simulink subsystem "AeroPropRef"  (R2024a)
settings: Solver=VariableStepAuto  StartTime=0.0  StopTime=10.0  RelTol=1e-3
undefined symbols (not defined in the file): Force_b, Fprop_r, H_b, Hdot_b, Moment_b, Mprop_r, SimIn, SimPar
libraries: starslibAxisTransformations x2, libAxisTransformations x2
settings Model: Creator=drhill  LastModifiedBy=azmol
settings SolverCC: AlgebraicLoopSolver=TrustRegion
settings OptimizationCC: ReuseModelBlockBuffer=off
settings DebuggingCC: UnconnectedInputMsg=warning  UnconnectedOutputMsg=warning  UnconnectedLineMsg=warning
settings ModelReferenceCC: EnableRefExpFcnMdlSchedulingChecks=on
settings RTWCC: GPUComputeCapability=3.5  DLArmComputeVersion=19.05

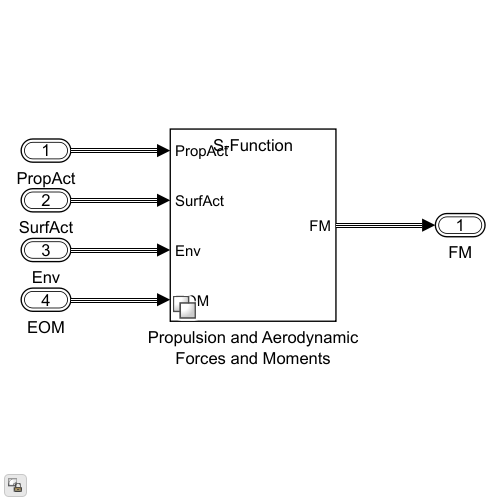
[thumbnail: Simulink's stored preview of the top-level diagram]
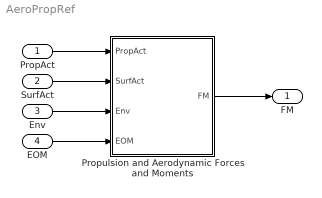
== system AeroPropRef ==
  PropAct : Inport  OutDataTypeStr=Bus: BUS_PROP_ACTUATOR
  SurfAct : Inport  Port=2  OutDataTypeStr=Bus: BUS_SURF_ACTUATOR
  Env : Inport  Port=3  OutDataTypeStr=Bus: EnvironmentBus
  EOM : Inport  Port=4  OutDataTypeStr=Bus: EomBus
  Propulsion and Aerodynamic Forces and Moments : Subsystem  Variant=on  VariantControl=Variant1
  FM : Outport  OutDataTypeStr=Bus: ForceMomentBus
  wires:
  Propulsion and Aerodynamic Forces and Moments/1(FM) -> FM/1
  Env/1 -> Propulsion and Aerodynamic Forces and Moments/3(Env)
  SurfAct/1 -> Propulsion and Aerodynamic Forces and Moments/2(SurfAct)
  PropAct/1 -> Propulsion and Aerodynamic Forces and Moments/1(PropAct)
  EOM/1 -> Propulsion and Aerodynamic Forces and Moments/4(EOM)

== system AeroPropRef/Propulsion and Aerodynamic Forces and Moments ==
  PropAct : Inport  OutDataTypeStr=Bus: BUS_PROP_ACTUATOR
  SurfAct : Inport  Port=2  OutDataTypeStr=Bus: BUS_SURF_ACTUATOR
  Env : Inport  Port=3  OutDataTypeStr=Bus: EnvironmentBus
  EOM : Inport  Port=4  OutDataTypeStr=Bus: EomBus
  Polynomial : Subsystem  VariantControl=GVS_FM_TYPE_POLYNOMIAL
  S-Function : Subsystem  VariantControl=GVS_FM_TYPE_SFUNCTION
  FM : Outport  OutDataTypeStr=Bus: ForceMomentBus

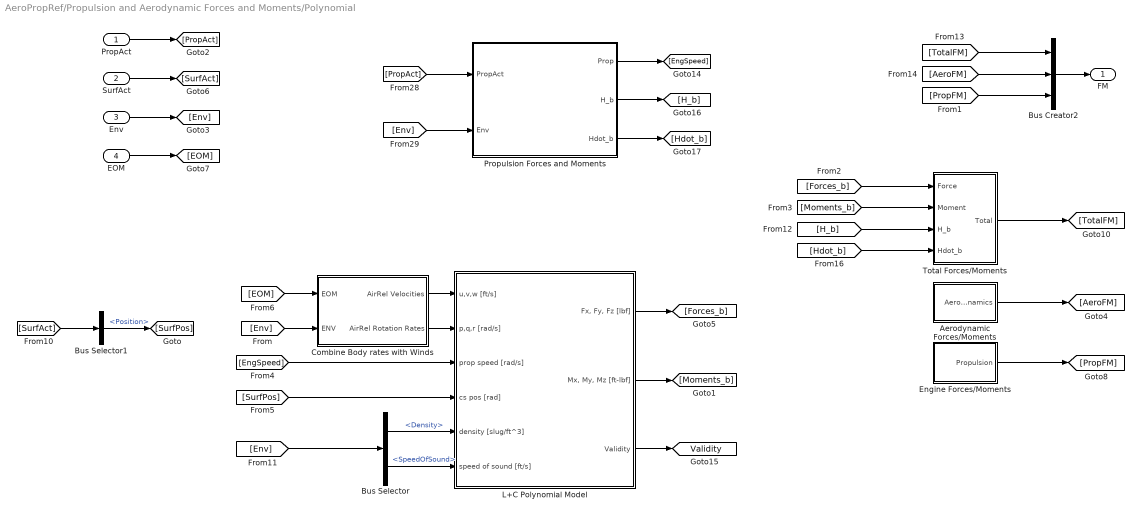
== system AeroPropRef/Propulsion and Aerodynamic Forces and Moments/Polynomial ==
  PropAct : Inport  OutDataTypeStr=Bus: BUS_PROP_ACTUATOR
  SurfAct : Inport  Port=2  OutDataTypeStr=Bus: BUS_SURF_ACTUATOR
  Env : Inport  Port=3  OutDataTypeStr=Bus: EnvironmentBus
  EOM : Inport  Port=4  OutDataTypeStr=Bus: EomBus
  Aerodynamic Forces/Moments : Subsystem
  Bus Creator2 : BusCreator  Inputs=3  OutDataTypeStr=Bus: ForceMomentBus
  Bus Selector : BusSelector  OutputSignals=Atmosphere.Density,Atmosphere.SpeedOfSound
  Bus Selector1 : BusSelector  OutputSignals=Position
  Combine Body rates with Winds : Subsystem
  Engine Forces/Moments : Subsystem
  L+C Polynomial Model : Subsystem  VariantControl=AeroModel == gncAeroModel.GGA  mask{Model=SimIn.Model, Units=SimIn.Units}
      mask prompts: Model "Model Parameters"; Units "Unit Conversions"
  Propulsion Forces and Moments : Subsystem  VariantControl=GVS_PROP_TYPE_NONE
  Total Forces/Moments : Subsystem
  FM : Outport  OutDataTypeStr=Bus: ForceMomentBus  VectorParamsAs1DForOutWhenUnconnected=off
  tag scope: Validity=global
  wires:
  L+C Polynomial Model/3(Validity) -> [Validity]
  Bus Selector/1 -> L+C Polynomial Model/5(density [slug/ft^3])  "<Density>"
  [Env] -> Bus Selector/1
  [EngSpeed] -> L+C Polynomial Model/3(prop speed [rad/s])
  L+C Polynomial Model/1("Fx, Fy, Fz [lbf]") -> [Forces_b]
  [SurfPos] -> L+C Polynomial Model/4(cs pos [rad])
  L+C Polynomial Model/2("Mx, My, Mz [ft-lbf]") -> [Moments_b]
  Propulsion Forces and Moments/1(Prop) -> [EngSpeed]
  [H_b] -> Total Forces/Moments/3(H_b)
  [Env] -> Propulsion Forces and Moments/2(Env)
  [PropAct] -> Propulsion Forces and Moments/1(PropAct)
  [PropFM] -> Bus Creator2/3
  [AeroFM] -> Bus Creator2/2
  [TotalFM] -> Bus Creator2/1
  Propulsion Forces and Moments/2(H_b) -> [H_b]
  Propulsion Forces and Moments/3(Hdot_b) -> [Hdot_b]
  PropAct/1 -> [PropAct]
  Env/1 -> [Env]
  EOM/1 -> [EOM]
  SurfAct/1 -> [SurfAct]
  [SurfAct] -> Bus Selector1/1
  Bus Selector1/1 -> [SurfPos]  "<Position>"
  Bus Creator2/1 -> FM/1
  Aerodynamic Forces/Moments/1(Aerodynamics) -> [AeroFM]
  Engine Forces/Moments/1(Propulsion) -> [PropFM]
  Bus Selector/2 -> L+C Polynomial Model/6(speed of sound [ft/s])  "<SpeedOfSound>"
  Combine Body rates with Winds/1(AirRel Velocities) -> L+C Polynomial Model/1(u,v,w [ft/s])
  [EOM] -> Combine Body rates with Winds/1(EOM)
  [Env] -> Combine Body rates with Winds/2(ENV)
  [Forces_b] -> Total Forces/Moments/1(Force)
  [Moments_b] -> Total Forces/Moments/2(Moment)
  [Hdot_b] -> Total Forces/Moments/4(Hdot_b)
  Total Forces/Moments/1(Total) -> [TotalFM]
  Combine Body rates with Winds/2(AirRel Rotation Rates) -> L+C Polynomial Model/2(p,q,r [rad/s])

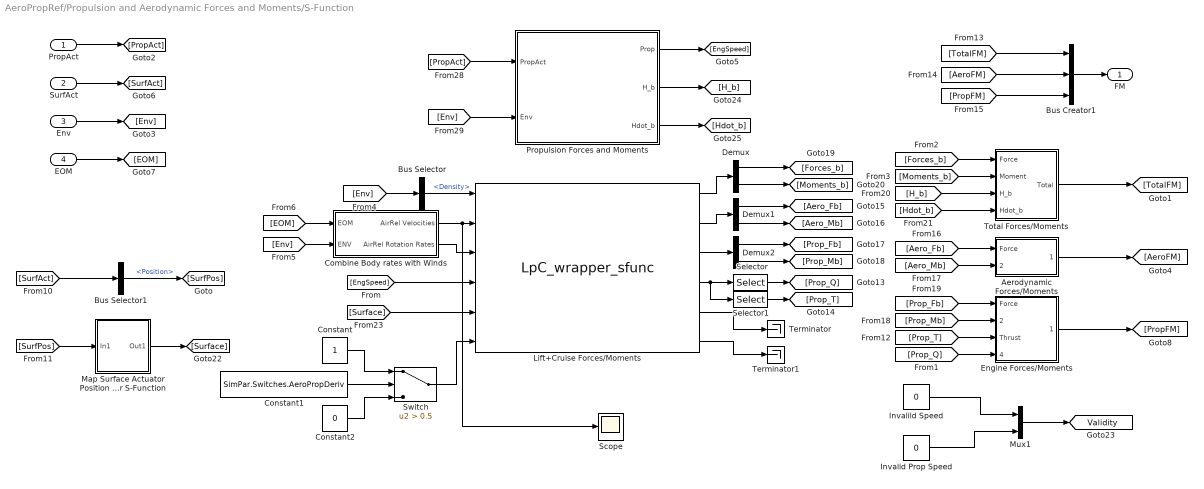
== system AeroPropRef/Propulsion and Aerodynamic Forces and Moments/S-Function ==
  PropAct : Inport  OutDataTypeStr=Bus: BUS_PROP_ACTUATOR
  SurfAct : Inport  Port=2  OutDataTypeStr=Bus: BUS_SURF_ACTUATOR
  Env : Inport  Port=3  OutDataTypeStr=Bus: EnvironmentBus
  EOM : Inport  Port=4  OutDataTypeStr=Bus: EomBus
  Aerodynamic Forces/Moments : Subsystem
  Bus Creator1 : BusCreator  Inputs=3  OutDataTypeStr=Bus: ForceMomentBus
  Bus Selector : BusSelector  OutputSignals=Atmosphere.Density
  Bus Selector1 : BusSelector  OutputSignals=Position
  Combine Body rates with Winds : Subsystem
  Constant : Constant
  Constant1 : Constant  Value=SimPar.Switches.AeroPropDeriv
  Constant2 : Constant  Value=0
  Demux : Demux  Outputs=[3 3]
  Demux1 : Demux  Outputs=[3 3]
  Demux2 : Demux  Outputs=[3 3]
  Engine Forces/Moments : Subsystem
  Invalid Prop Speed : Constant  Value=0
  Invalild Speed : Constant  Value=0
  Lift+Cruise Forces/Moments : S-Function  FunctionName=LpC_wrapper_sfunc  SFunctionDeploymentMode=off  EnableBusSupport=off
      mask Display:
      | port_label('input',1,'air density');
      | port_label('input',2,'Velocity, body');
      | port_label('input',3,'Angular Rates, body');
      | port_label('input',4,'Engine Speeds');
      | port_label('input',5,'Surface Deflections');
      | port_label('input',6,'Compute Derivatives');
      | port_label('output',1,'Total Forces/Moments');
      | port_label('output',2,'Aero Total Forces/Moments');
      | port_label('output',3,'Prop Forces/Moments');
      | port_label('output',4,'Prop Torque/Thrust');
      | port_label('output',5,'FM_x');
      | port_label('output',6,'FM_u');
  Map Surface Actuator Position To Surface Inputs for S-Function : Subsystem
  Mux1 : Mux  Inputs=2
  Propulsion Forces and Moments : Subsystem  VariantControl=GVS_PROP_TYPE_NONE
  Scope : Scope
  Selector : Selector  NumberOfDimensions=2  InputPortWidth=3  IndexOptions=Index vector (dialog),Select all  Indices=1,1  OutputSizes=1,1
  Selector1 : Selector  NumberOfDimensions=2  InputPortWidth=3  IndexOptions=Index vector (dialog),Select all  Indices=2,1  OutputSizes=1,1
  Switch : Switch  Criteria=u2 > Threshold  Threshold=0.5  OutDataTypeStr=boolean  SaturateOnIntegerOverflow=off  InputSameDT=off
  Terminator : Terminator
  Terminator1 : Terminator
  Total Forces/Moments : Subsystem
  FM : Outport  OutDataTypeStr=Bus: ForceMomentBus  VectorParamsAs1DForOutWhenUnconnected=off
  tag scope: Validity=global
  wires:
  PropAct/1 -> [PropAct]
  Env/1 -> [Env]
  EOM/1 -> [EOM]
  SurfAct/1 -> [SurfAct]
  [EngSpeed] -> Lift+Cruise Forces/Moments/4
  Constant2/1 -> Switch/3
  [Surface] -> Lift+Cruise Forces/Moments/5
  Constant/1 -> Switch/1
  [Env] -> Bus Selector/1
  Bus Selector/1 -> Lift+Cruise Forces/Moments/1  "<Density>"
  Propulsion Forces and Moments/3(Hdot_b) -> [Hdot_b]
  [EOM] -> Combine Body rates with Winds/1(EOM)
  Propulsion Forces and Moments/2(H_b) -> [H_b]
  Lift+Cruise Forces/Moments/5 -> Terminator/1
  Propulsion Forces and Moments/1(Prop) -> [EngSpeed]
  [PropAct] -> Propulsion Forces and Moments/1(PropAct)
  [Env] -> Propulsion Forces and Moments/2(Env)
  [SurfAct] -> Bus Selector1/1
  Bus Selector1/1 -> [SurfPos]  "<Position>"
  Bus Creator1/1 -> FM/1
  [TotalFM] -> Bus Creator1/1
  [AeroFM] -> Bus Creator1/2
  [PropFM] -> Bus Creator1/3
  Total Forces/Moments/1(Total) -> [TotalFM]
  Aerodynamic Forces/Moments/1(Aerodynamics) -> [AeroFM]
  Engine Forces/Moments/1(Propulsion) -> [PropFM]
  [Moments_b] -> Total Forces/Moments/2(Moment)
  [Forces_b] -> Total Forces/Moments/1(Force)
  [SurfPos] -> Map Surface Actuator Position To Surface Inputs for S-Function/1(In1)
  Map Surface Actuator Position To Surface Inputs for S-Function/1(Out1) -> [Surface]
  [Prop_Q] -> Engine Forces/Moments/4(Torque)
  [Prop_T] -> Engine Forces/Moments/3(Thrust)
  Lift+Cruise Forces/Moments/6 -> Terminator1/1
  Lift+Cruise Forces/Moments/1 -> Demux/1
  Lift+Cruise Forces/Moments/2 -> Demux1/1
  Lift+Cruise Forces/Moments/3 -> Demux2/1
  Demux/1 -> [Forces_b]
  Demux/2 -> [Moments_b]
  Selector1/1 -> [Prop_T]
  Selector/1 -> [Prop_Q]
  Demux1/1 -> [Aero_Fb]
  Demux1/2 -> [Aero_Mb]
  Demux2/1 -> [Prop_Fb]
  Demux2/2 -> [Prop_Mb]
  [Prop_Fb] -> Engine Forces/Moments/1(Force)
  [Prop_Mb] -> Engine Forces/Moments/2(Moment)
  [Aero_Fb] -> Aerodynamic Forces/Moments/1(Force)
  [Aero_Mb] -> Aerodynamic Forces/Moments/2(Moment)
  Mux1/1 -> [Validity]
  Invalild Speed/1 -> Mux1/1
  Invalid Prop Speed/1 -> Mux1/2
  Constant1/1 -> Switch/2
  [Env] -> Combine Body rates with Winds/2(ENV)
  Lift+Cruise Forces/Moments/4 -> Selector1/1, Selector/1
  Combine Body rates with Winds/1(AirRel Velocities) -> Lift+Cruise Forces/Moments/2, Scope/1
  Combine Body rates with Winds/2(AirRel Rotation Rates) -> Lift+Cruise Forces/Moments/3
  Switch/1 -> Lift+Cruise Forces/Moments/6
  [H_b] -> Total Forces/Moments/3(H_b)
  [Hdot_b] -> Total Forces/Moments/4(Hdot_b)

== system AeroPropRef/Propulsion and Aerodynamic Forces and Moments/Polynomial/Aerodynamic Forces//Moments ==
  RenameAeroForceMomentBus : Subsystem
  Aerodynamics : Outport
  wires:
  RenameAeroForceMomentBus/1(Aerodynamics) -> Aerodynamics/1

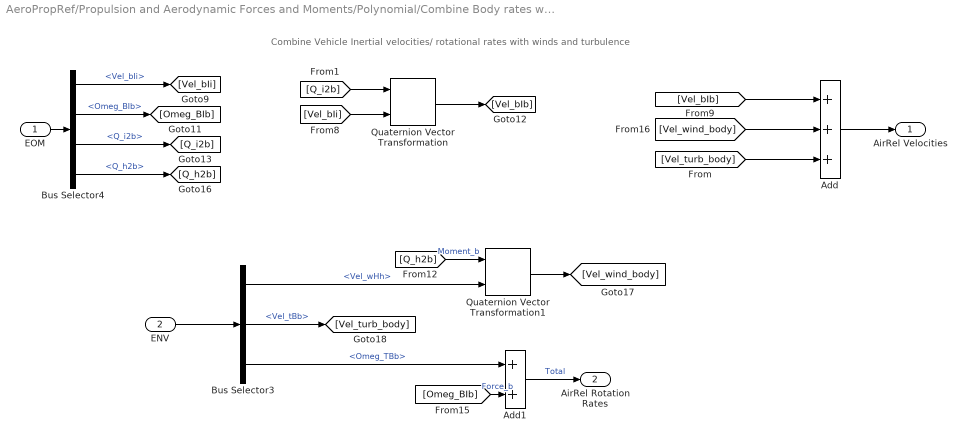
== system AeroPropRef/Propulsion and Aerodynamic Forces and Moments/Polynomial/Combine Body rates with Winds ==
  note: Combine Vehicle Inertial velocities/ rotational rates with winds and turbulence
  EOM : Inport
  ENV : Inport  Port=2
  Add : Sum  Inputs=+++
  Add1 : Sum
  Bus Selector3 : BusSelector  OutputSignals=Wind.Vel_wHh,Turbulence.Vel_tBb,Turbulence.Omeg_TBb
  Bus Selector4 : BusSelector  OutputSignals=InertialData.Vel_bIi,InertialData.Omeg_BIb,InertialData.Q_i2b,WorldRelativeData.Q_h2b
  Quaternion Vector Transformation : starslibAxisTransformations/Quaternion Vector Transformation  n=0
  Quaternion Vector Transformation1 : starslibAxisTransformations/Quaternion Vector Transformation  n=0
  AirRel Velocities : Outport
  AirRel Rotation Rates : Outport  Port=2
  wires:
  [Q_h2b] -> Quaternion Vector Transformation1/1  "Moment_b"
  [Omeg_BIb] -> Add1/2  "Force_b"
  Add1/1 -> AirRel Rotation Rates/1  "Total"
  Add/1 -> AirRel Velocities/1
  Bus Selector3/3 -> Add1/1  "<Omeg_TBb>"
  Bus Selector3/2 -> [Vel_turb_body]  "<Vel_tBb>"
  Bus Selector4/2 -> [Omeg_BIb]  "<Omeg_BIb>"
  Bus Selector4/3 -> [Q_i2b]  "<Q_i2b>"
  Bus Selector4/4 -> [Q_h2b]  "<Q_h2b>"
  Bus Selector4/1 -> [Vel_bIi]  "<Vel_bIi>"
  ENV/1 -> Bus Selector3/1
  EOM/1 -> Bus Selector4/1
  [Vel_wind_body] -> Add/2
  [Vel_bIi] -> Quaternion Vector Transformation/2
  [Vel_bIb] -> Add/1
  [Vel_turb_body] -> Add/3
  [Q_i2b] -> Quaternion Vector Transformation/1
  Bus Selector3/1 -> Quaternion Vector Transformation1/2  "<Vel_wHh>"
  Quaternion Vector Transformation1/1 -> [Vel_wind_body]
  Quaternion Vector Transformation/1 -> [Vel_bIb]

== system AeroPropRef/Propulsion and Aerodynamic Forces and Moments/Polynomial/Engine Forces//Moments ==
  RenameEngineForceMomentBus : Subsystem
  Propulsion : Outport
  wires:
  RenameEngineForceMomentBus/1(Propulsion) -> Propulsion/1

== system AeroPropRef/Propulsion and Aerodynamic Forces and Moments/Polynomial/L+C Polynomial Model ==
  note: Control surface positions
      | 1-2: L,R Aileron
      | 3-4: L,R Elevator
      | 5: Rudder
  note: controls
  note: states
  note: atmosphere
  u,v,w [ft/s] : Inport
  p,q,r [rad/s] : Inport  Port=2
  prop speed [rad/s] : Inport  Port=3
  cs pos [rad] : Inport  Port=4
  density [slug/ft^3] : Inport  Port=5
  speed of sound [ft/s] : Inport  Port=6
  Data Type Conversion : DataTypeConversion  SaturateOnIntegerOverflow=off  RndMeth=Floor
  L+C Aerodynamic Model : MATLAB Function  TreatAsAtomicUnit=on
  Mux : Mux  Inputs=2
  "Fx, Fy, Fz [lbf]" : Outport
  "Mx, My, Mz [ft-lbf]" : Outport  Port=2
  Validity : Outport  Port=3  OutDataTypeStr=double  PortDimensions=[1 2]
  wires:
  Data Type Conversion/1 -> Validity/1
  speed of sound [ft/s]/1 -> L+C Aerodynamic Model/5(a)
  L+C Aerodynamic Model/3(Validity) -> Data Type Conversion/1
  Mux/1 -> L+C Aerodynamic Model/1(x)
  cs pos [rad]/1 -> L+C Aerodynamic Model/3(d)
  prop speed [rad/s]/1 -> L+C Aerodynamic Model/2(n)
  p,q,r [rad/s]/1 -> Mux/2
  u,v,w [ft/s]/1 -> Mux/1
  L+C Aerodynamic Model/1(Fb) -> "Fx, Fy, Fz [lbf]"/1
  L+C Aerodynamic Model/2(Mb) -> "Mx, My, Mz [ft-lbf]"/1
  density [slug/ft^3]/1 -> L+C Aerodynamic Model/4(rho)

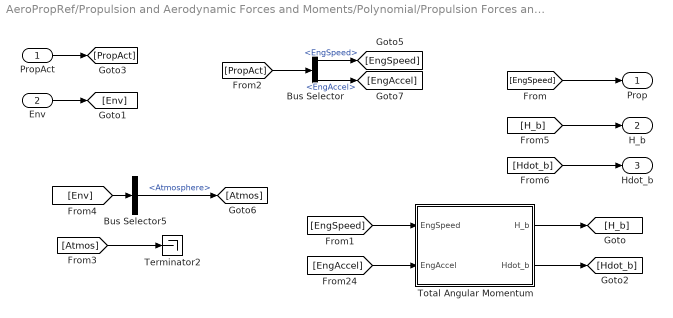
== system AeroPropRef/Propulsion and Aerodynamic Forces and Moments/Polynomial/Propulsion Forces and Moments ==
  PropAct : Inport
  Env : Inport  Port=2
  Bus Selector : BusSelector  OutputSignals=EngSpeed,EngAccel
  Bus Selector5 : BusSelector  OutputSignals=Atmosphere
  Terminator2 : Terminator
  Total Angular Momentum : Subsystem  mask{Model=SimIn.Model}
      mask prompts: Model "Modeling Parameters"
  Prop : Outport  VectorParamsAs1DForOutWhenUnconnected=off
  H_b : Outport  Port=2  VectorParamsAs1DForOutWhenUnconnected=off
  Hdot_b : Outport  Port=3  VectorParamsAs1DForOutWhenUnconnected=off
  wires:
  [Atmos] -> Terminator2/1
  [EngSpeed] -> Prop/1
  Env/1 -> [Env]
  PropAct/1 -> [PropAct]
  Bus Selector5/1 -> [Atmos]  "<Atmosphere>"
  Bus Selector/1 -> [EngSpeed]  "<EngSpeed>"
  Bus Selector/2 -> [EngAccel]  "<EngAccel>"
  [PropAct] -> Bus Selector/1
  [Env] -> Bus Selector5/1
  [EngAccel] -> Total Angular Momentum/2(EngAccel)
  [EngSpeed] -> Total Angular Momentum/1(EngSpeed)
  Total Angular Momentum/1(H_b) -> [H_b]
  Total Angular Momentum/2(Hdot_b) -> [Hdot_b]
  [H_b] -> H_b/1
  [Hdot_b] -> Hdot_b/1

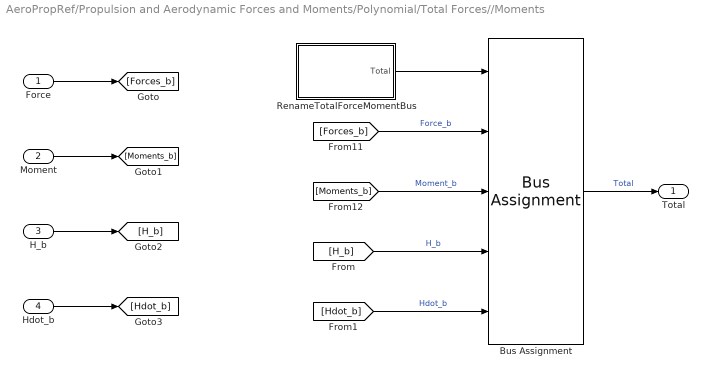
== system AeroPropRef/Propulsion and Aerodynamic Forces and Moments/Polynomial/Total Forces//Moments ==
  Force : Inport
  Moment : Inport  Port=2
  H_b : Inport  Port=3
  Hdot_b : Inport  Port=4
  Bus Assignment : BusAssignment  AssignedSignals=Force_b,Moment_b,H_b,Hdot_b
  RenameTotalForceMomentBus : Subsystem
  Total : Outport
  wires:
  [H_b] -> Bus Assignment/4  "H_b"
  [Hdot_b] -> Bus Assignment/5  "Hdot_b"
  H_b/1 -> [H_b]
  Hdot_b/1 -> [Hdot_b]
  [Moments_b] -> Bus Assignment/3  "Moment_b"
  RenameTotalForceMomentBus/1(Total) -> Bus Assignment/1
  [Forces_b] -> Bus Assignment/2  "Force_b"
  Bus Assignment/1 -> Total/1  "Total"
  Moment/1 -> [Moments_b]
  Force/1 -> [Forces_b]

== system AeroPropRef/Propulsion and Aerodynamic Forces and Moments/S-Function/Aerodynamic Forces//Moments ==
  Force : Inport
  Moment : Inport  Port=2
  Bus Assignment : BusAssignment  AssignedSignals=Force_b,Moment_b
  RenameAeroForceMomentBus : Subsystem
  Aerodynamics : Outport
  wires:
  Force/1 -> [Aero_Fb]
  Moment/1 -> [Aero_Mb]
  RenameAeroForceMomentBus/1(Aerodynamics) -> Bus Assignment/1
  [Aero_Fb] -> Bus Assignment/2
  [Aero_Mb] -> Bus Assignment/3
  Bus Assignment/1 -> Aerodynamics/1  "Aerodynamics"

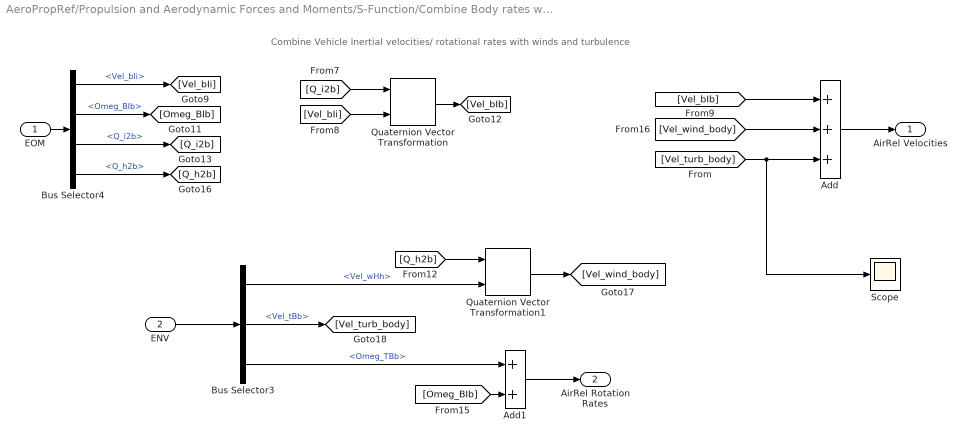
== system AeroPropRef/Propulsion and Aerodynamic Forces and Moments/S-Function/Combine Body rates with Winds ==
  note: Combine Vehicle Inertial velocities/ rotational rates with winds and turbulence
  EOM : Inport
  ENV : Inport  Port=2
  Add : Sum  Inputs=+++
  Add1 : Sum
  Bus Selector3 : BusSelector  OutputSignals=Wind.Vel_wHh,Turbulence.Vel_tBb,Turbulence.Omeg_TBb
  Bus Selector4 : BusSelector  OutputSignals=InertialData.Vel_bIi,InertialData.Omeg_BIb,InertialData.Q_i2b,WorldRelativeData.Q_h2b
  Quaternion Vector Transformation : libAxisTransformations/Quaternion Vector Transformation  n=0
  Quaternion Vector Transformation1 : libAxisTransformations/Quaternion Vector Transformation  n=0
  Scope : Scope
  AirRel Velocities : Outport
  AirRel Rotation Rates : Outport  Port=2
  wires:
  [Vel_wind_body] -> Add/2
  [Vel_turb_body] -> Add/3, Scope/1
  EOM/1 -> Bus Selector4/1
  Quaternion Vector Transformation1/1 -> [Vel_wind_body]
  ENV/1 -> Bus Selector3/1
  Bus Selector3/2 -> [Vel_turb_body]  "<Vel_tBb>"
  [Q_i2b] -> Quaternion Vector Transformation/1
  Bus Selector3/3 -> Add1/1  "<Omeg_TBb>"
  Quaternion Vector Transformation/1 -> [Vel_bIb]
  Bus Selector3/1 -> Quaternion Vector Transformation1/2  "<Vel_wHh>"
  Bus Selector4/4 -> [Q_h2b]  "<Q_h2b>"
  [Q_h2b] -> Quaternion Vector Transformation1/1
  [Vel_bIi] -> Quaternion Vector Transformation/2
  [Vel_bIb] -> Add/1
  [Omeg_BIb] -> Add1/2
  Bus Selector4/3 -> [Q_i2b]  "<Q_i2b>"
  Add1/1 -> AirRel Rotation Rates/1
  Bus Selector4/1 -> [Vel_bIi]  "<Vel_bIi>"
  Bus Selector4/2 -> [Omeg_BIb]  "<Omeg_BIb>"
  Add/1 -> AirRel Velocities/1

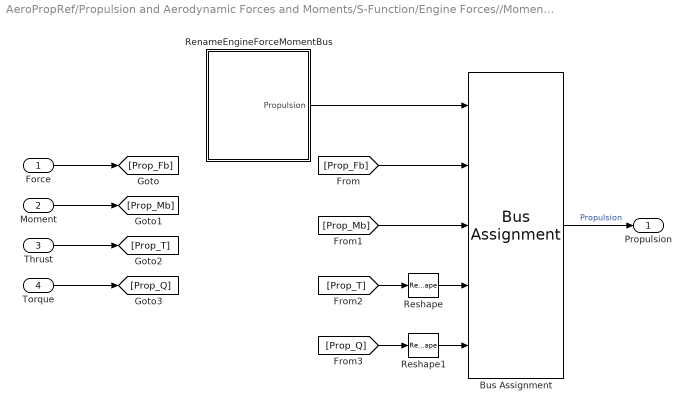
== system AeroPropRef/Propulsion and Aerodynamic Forces and Moments/S-Function/Engine Forces//Moments ==
  Force : Inport
  Moment : Inport  Port=2
  Thrust : Inport  Port=3
  Torque : Inport  Port=4
  Bus Assignment : BusAssignment  AssignedSignals=Force_b,Moment_b,Fprop_r,Mprop_r
  RenameEngineForceMomentBus : Subsystem
  Reshape : Reshape
  Reshape1 : Reshape
  Propulsion : Outport
  wires:
  Moment/1 -> [Prop_Mb]
  RenameEngineForceMomentBus/1(Propulsion) -> Bus Assignment/1
  Bus Assignment/1 -> Propulsion/1  "Propulsion"
  [Prop_Fb] -> Bus Assignment/2
  Force/1 -> [Prop_Fb]
  [Prop_Mb] -> Bus Assignment/3
  Thrust/1 -> [Prop_T]
  Torque/1 -> [Prop_Q]
  [Prop_T] -> Reshape/1
  [Prop_Q] -> Reshape1/1
  Reshape/1 -> Bus Assignment/4
  Reshape1/1 -> Bus Assignment/5

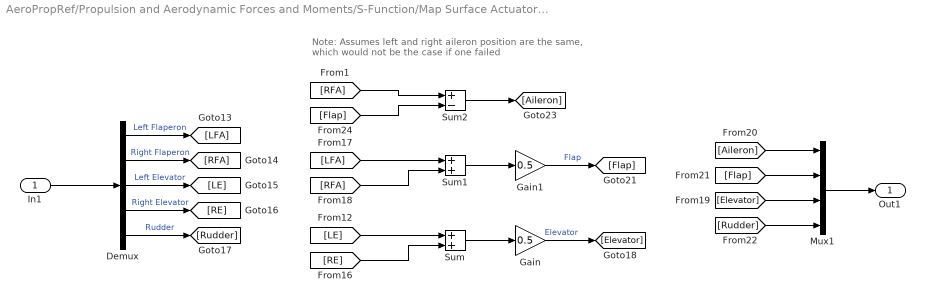
== system AeroPropRef/Propulsion and Aerodynamic Forces and Moments/S-Function/Map Surface Actuator Position To Surface Inputs for S-Function ==
  note: Note:  Assumes left and right aileron position are the same,
      |           which would not be the case if one failed
  In1 : Inport
  Demux : Demux  Outputs=SimIn.numSurfaces
  Gain : Gain  Gain=0.5
  Gain1 : Gain  Gain=0.5
  Mux1 : Mux
  Sum : Sum
  Sum1 : Sum
  Sum2 : Sum  Inputs=+-
  Out1 : Outport
  wires:
  Gain1/1 -> [Flap]  "Flap"
  [Elevator] -> Mux1/3
  [LE] -> Sum/1
  [Flap] -> Mux1/2
  [RFA] -> Sum2/1
  Demux/1 -> [LFA]  "Left Flaperon"
  Mux1/1 -> Out1/1
  [RFA] -> Sum1/2
  Demux/2 -> [RFA]  "Right Flaperon"
  Demux/5 -> [Rudder]  "Rudder"
  [Aileron] -> Mux1/1
  [Rudder] -> Mux1/4
  Gain/1 -> [Elevator]  "Elevator"
  Demux/4 -> [RE]  "Right Elevator"
  Sum2/1 -> [Aileron]
  Sum1/1 -> Gain1/1
  [LFA] -> Sum1/1
  Demux/3 -> [LE]  "Left Elevator"
  [RE] -> Sum/2
  Sum/1 -> Gain/1
  [Flap] -> Sum2/2
  In1/1 -> Demux/1

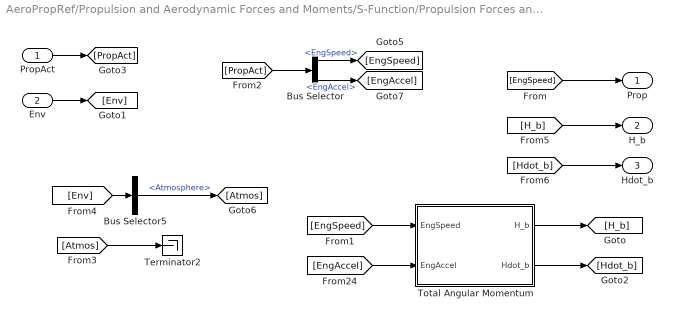
== system AeroPropRef/Propulsion and Aerodynamic Forces and Moments/S-Function/Propulsion Forces and Moments ==
  PropAct : Inport
  Env : Inport  Port=2
  Bus Selector : BusSelector  OutputSignals=EngSpeed,EngAccel
  Bus Selector5 : BusSelector  OutputSignals=Atmosphere
  Terminator2 : Terminator
  Total Angular Momentum : Subsystem  mask{Model=SimIn.CModel}
      mask prompts: Model "Modeling Parameters"
  Prop : Outport  VectorParamsAs1DForOutWhenUnconnected=off
  H_b : Outport  Port=2  VectorParamsAs1DForOutWhenUnconnected=off
  Hdot_b : Outport  Port=3  VectorParamsAs1DForOutWhenUnconnected=off
  wires:
  PropAct/1 -> [PropAct]
  Env/1 -> [Env]
  [EngSpeed] -> Prop/1
  [Atmos] -> Terminator2/1
  Bus Selector5/1 -> [Atmos]  "<Atmosphere>"
  Bus Selector/1 -> [EngSpeed]  "<EngSpeed>"
  Bus Selector/2 -> [EngAccel]  "<EngAccel>"
  [PropAct] -> Bus Selector/1
  [Env] -> Bus Selector5/1
  [EngAccel] -> Total Angular Momentum/2(EngAccel)
  [EngSpeed] -> Total Angular Momentum/1(EngSpeed)
  Total Angular Momentum/1(H_b) -> [H_b]
  Total Angular Momentum/2(Hdot_b) -> [Hdot_b]
  [H_b] -> H_b/1
  [Hdot_b] -> Hdot_b/1

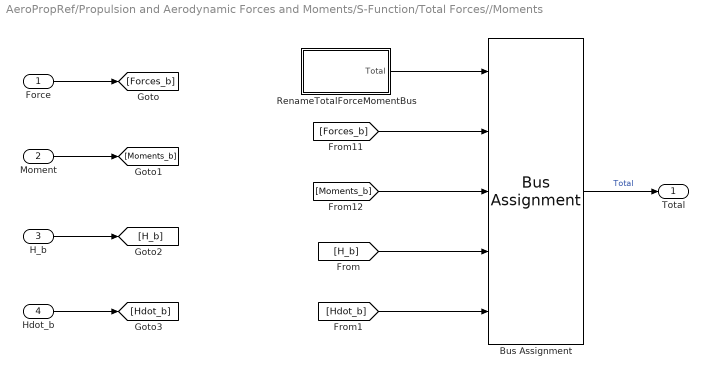
== system AeroPropRef/Propulsion and Aerodynamic Forces and Moments/S-Function/Total Forces//Moments ==
  Force : Inport
  Moment : Inport  Port=2
  H_b : Inport  Port=3
  Hdot_b : Inport  Port=4
  Bus Assignment : BusAssignment  AssignedSignals=Force_b,Moment_b,H_b,Hdot_b
  RenameTotalForceMomentBus : Subsystem
  Total : Outport
  wires:
  RenameTotalForceMomentBus/1(Total) -> Bus Assignment/1
  Bus Assignment/1 -> Total/1  "Total"
  Moment/1 -> [Moments_b]
  Force/1 -> [Forces_b]
  [Forces_b] -> Bus Assignment/2
  [Moments_b] -> Bus Assignment/3
  [Hdot_b] -> Bus Assignment/5
  [H_b] -> Bus Assignment/4
  H_b/1 -> [H_b]
  Hdot_b/1 -> [Hdot_b]

== system AeroPropRef/Propulsion and Aerodynamic Forces and Moments/Polynomial/Aerodynamic Forces//Moments/RenameAeroForceMomentBus ==
  Bus Creator2 : BusCreator  Inputs=2  OutDataTypeStr=Bus: AeroFMBus
  Constant2 : Constant  Value=zeros(3,1)
  Constant3 : Constant  Value=zeros(3,1)
  Aerodynamics : Outport
  wires:
  Constant3/1 -> Bus Creator2/2  "Moment_b"
  Constant2/1 -> Bus Creator2/1  "Force_b"
  Bus Creator2/1 -> Aerodynamics/1  "Aerodynamics"

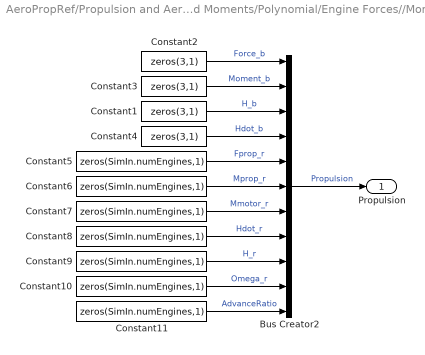
== system AeroPropRef/Propulsion and Aerodynamic Forces and Moments/Polynomial/Engine Forces//Moments/RenameEngineForceMomentBus ==
  Bus Creator2 : BusCreator  Inputs=11  OutDataTypeStr=Bus: EngineFMBus
  Constant{1..4} (4 alike) : Constant  Value=zeros(3,1)
  Constant{5..11} (7 alike) : Constant  Value=zeros(SimIn.numEngines,1)
  Propulsion : Outport
  wires:
  Constant3/1 -> Bus Creator2/2  "Moment_b"
  Constant2/1 -> Bus Creator2/1  "Force_b"
  Bus Creator2/1 -> Propulsion/1  "Propulsion"
  Constant1/1 -> Bus Creator2/3  "H_b"
  Constant4/1 -> Bus Creator2/4  "Hdot_b"
  Constant5/1 -> Bus Creator2/5  "Fprop_r"
  Constant6/1 -> Bus Creator2/6  "Mprop_r"
  Constant7/1 -> Bus Creator2/7  "Mmotor_r"
  Constant8/1 -> Bus Creator2/8  "Hdot_r"
  Constant9/1 -> Bus Creator2/9  "H_r"
  Constant10/1 -> Bus Creator2/10  "Omega_r"
  Constant11/1 -> Bus Creator2/11  "AdvanceRatio"

== system AeroPropRef/Propulsion and Aerodynamic Forces and Moments/Polynomial/Propulsion Forces and Moments/Total Angular Momentum ==
  EngSpeed : Inport
  EngAccel : Inport  Port=2
  MATLAB Function : MATLAB Function  TreatAsAtomicUnit=on
  H_b : Outport
  Hdot_b : Outport  Port=2
  wires:
  MATLAB Function/2(Hdot_b) -> Hdot_b/1
  MATLAB Function/1(H_b) -> H_b/1
  EngAccel/1 -> MATLAB Function/2(EngAccel)
  EngSpeed/1 -> MATLAB Function/1(EngSpeed)

== system AeroPropRef/Propulsion and Aerodynamic Forces and Moments/Polynomial/Total Forces//Moments/RenameTotalForceMomentBus ==
  Bus Creator2 : BusCreator  Inputs=4  OutDataTypeStr=Bus: TotalFMBus
  Constant{2..5} (4 alike) : Constant  Value=zeros(3,1)
  Total : Outport
  wires:
  Constant3/1 -> Bus Creator2/2  "Moment_b"
  Constant4/1 -> Bus Creator2/3  "H_b"
  Constant2/1 -> Bus Creator2/1  "Force_b"
  Constant5/1 -> Bus Creator2/4  "Hdot_b"
  Bus Creator2/1 -> Total/1  "Total"

== system AeroPropRef/Propulsion and Aerodynamic Forces and Moments/S-Function/Aerodynamic Forces//Moments/RenameAeroForceMomentBus ==
  Bus Creator2 : BusCreator  Inputs=2  OutDataTypeStr=Bus: AeroFMBus
  Constant2 : Constant  Value=zeros(3,1)
  Constant3 : Constant  Value=zeros(3,1)
  Aerodynamics : Outport
  wires:
  Constant3/1 -> Bus Creator2/2  "Moment_b"
  Constant2/1 -> Bus Creator2/1  "Force_b"
  Bus Creator2/1 -> Aerodynamics/1  "Aerodynamics"

== system AeroPropRef/Propulsion and Aerodynamic Forces and Moments/S-Function/Engine Forces//Moments/RenameEngineForceMomentBus ==
  Bus Creator2 : BusCreator  Inputs=11  OutDataTypeStr=Bus: EngineFMBus
  Constant{1..4} (4 alike) : Constant  Value=zeros(3,1)
  Constant{5..11} (7 alike) : Constant  Value=zeros(1,SimIn.numEngines)
  Propulsion : Outport
  wires:
  Constant3/1 -> Bus Creator2/2  "Moment_b"
  Constant2/1 -> Bus Creator2/1  "Force_b"
  Bus Creator2/1 -> Propulsion/1  "Propulsion"
  Constant1/1 -> Bus Creator2/3  "H_b"
  Constant4/1 -> Bus Creator2/4  "Hdot_b"
  Constant7/1 -> Bus Creator2/7  "Mmotor_r"
  Constant8/1 -> Bus Creator2/8  "Hdot_r"
  Constant9/1 -> Bus Creator2/9  "H_r"
  Constant10/1 -> Bus Creator2/10  "Omega_r"
  Constant11/1 -> Bus Creator2/11  "AdvanceRatio"
  Constant5/1 -> Bus Creator2/5  "Fprop_r"
  Constant6/1 -> Bus Creator2/6  "Mprop_r"

== system AeroPropRef/Propulsion and Aerodynamic Forces and Moments/S-Function/Propulsion Forces and Moments/Total Angular Momentum ==
  EngSpeed : Inport
  EngAccel : Inport  Port=2
  MATLAB Function : MATLAB Function  TreatAsAtomicUnit=on
  H_b : Outport
  Hdot_b : Outport  Port=2
  wires:
  MATLAB Function/2(Hdot_b) -> Hdot_b/1
  MATLAB Function/1(H_b) -> H_b/1
  EngAccel/1 -> MATLAB Function/2(EngAccel)
  EngSpeed/1 -> MATLAB Function/1(EngSpeed)

== system AeroPropRef/Propulsion and Aerodynamic Forces and Moments/S-Function/Total Forces//Moments/RenameTotalForceMomentBus ==
  Bus Creator2 : BusCreator  Inputs=4  OutDataTypeStr=Bus: TotalFMBus
  Constant{2..5} (4 alike) : Constant  Value=zeros(3,1)
  Total : Outport
  wires:
  Bus Creator2/1 -> Total/1  "Total"
  Constant2/1 -> Bus Creator2/1  "Force_b"
  Constant3/1 -> Bus Creator2/2  "Moment_b"
  Constant4/1 -> Bus Creator2/3  "H_b"
  Constant5/1 -> Bus Creator2/4  "Hdot_b"

== matlab function AeroPropRef/Propulsion and Aerodynamic Forces and Moments/Polynomial/L+C Polynomial Model/L+C Aerodynamic Model ==
  data: x input; n input; d input; rho input; a input; Fb output; Units parameter; Mb output; Validity output; Model parameter
function [Fb,Mb,Validity] = run_LpC_aero(x,n,d,rho,a,Units,Model)
% run_LpC_aero - Implements the Lift+Cruise polynomial aero models
%
% DESCRIPTION: 
%   This script runs the polynomial aerodynamic models for Lift+Cruise
%
% INPUT: 
%   x - state vector containing body-axis velocity and body-axis angular 
%       rates, x=[u,v,w,p,q,r] in ft/s and rad/s
%   n - vector containing propeller speed values, n=[n1,n2...] in rad/s
%   d - vector contol surface positions, n=[d1,d2...] in rad
%   rho - atmosphereic density in slug/ft^3
%   a - speed of seound in ft/s
%   Units - SimIn.Units
%   Model - SimIn.Model
%
% OUTPUT:
%   Fb - body-axis aerodynamic forces in lbf
%   Mb - body-axis aerodynamic moments in ft-lbf
%
% WRITTEN BY:
%   Benjamin M. Simmons
%   NASA Langley Research Center
%   Email: benjamin.m.simmons@nasa.gov
%
% HISTORY:
%   February 12, 2020 - Created and debugged for Lift+Cruise, BMS
%   April 15, 2020 - Modified to call LA-8 model, BMS
%   April 27, 2020 - Updated function for L+C model, BMS
%   May 6, 2020 - Added blending capability for overlapping models, BMS
%   January 04, 2021 - Added density as an input for v2 aero models, BMS
%

Fb=zeros(3,1);Mb=zeros(3,1); 

% select blending method for combining overlapping models
% 1: linear blending
% 2: smooth "sigmoid-like" blending (continuous and differentiable)
% 3: smooth quintic transition polynomial blending (continuous and twice differentiable)
blending_method=3;


% call Lift+Cruise aero models

% % L+C version 1 aerodynamic models
% [X,Y,Z,L,M,N,Validity] = LpC_aero_p_v1(x,n,d,blending_method,c);

% L+C version 2 aerodynamic models
[X,Y,Z,L,M,N,Validity] = LpC_aero_p_v2(x,n,d,rho,a,blending_method,Units,Model);

% body-axis forces
Fb=[X;Y;Z];

% body-axis moments
Mb=[L;M;N];

end

== matlab function AeroPropRef/Propulsion and Aerodynamic Forces and Moments/Polynomial/Propulsion Forces and Moments/Total Angular Momentum/MATLAB Function ==
  data: EngSpeed input; H_b output; EngAccel input; Hdot_b output; Model parameter
function [H_b,Hdot_b] = total_angular_momentum(EngSpeed, EngAccel, Model)
% angular momentum of the rotating portion of the propulsion system
%
% DESCRIPTION: 
%   This function calculates the angular momentum and rate of angular
%   momentum components for the rotating portion of each propulsor. The
%   contributions from each propulsor are then summed to output the total
%   angular moment and angular momentum rate.
%
% INPUTS:
%   EngSpeed - Npx1 engine rotational speed [rad/s]
%   EngAccel - Npx1 engine rotational speed rate [rad/s^2]
%   Model - Model parameters
%
% OUTPUTS:
%   H_b - 3x1 total angular momentum in the body frame [slug-ft^2/s]
%   Hdot_b - 3x1 total angular momentum rate in the body frame [slug-ft^2/s^2]
%
% WRITTEN BY:
%   Benjamin M. Simmons
%   NASA Langley Research Center
%   Email: benjamin.m.simmons@nasa.gov
%
% HISTORY:
%   February 16, 2021 - Created and debugged, BMS
%

% propulsion inertia [slug-ft^2]
Ip=Model.Ip';

% unit vector of the propeller/rotor axis of rotation
p_rot_axis_e=Model.p_T_e;

% propeller/rotor rotation direction (CW=+1, CCW=-1)
Prop_dir=Model.prop_spin';

% hub frame angular momentum and angular momentum rate
H_h=EngSpeed.*Ip.*Prop_dir;
Hdot_h=EngAccel.*Ip.*Prop_dir;

% body frame angular momentum and angular momentum rate
H_b=p_rot_axis_e*H_h;
Hdot_b=p_rot_axis_e*Hdot_h;

% no angular momentum
% H_b=[0;0;0];
% Hdot_b=[0;0;0];

return

== matlab function AeroPropRef/Propulsion and Aerodynamic Forces and Moments/S-Function/Propulsion Forces and Moments/Total Angular Momentum/MATLAB Function ==
  data: EngSpeed input; H_b output; EngAccel input; Hdot_b output; Model parameter
function [H_b,Hdot_b] = total_angular_momentum(EngSpeed, EngAccel, Model)
% angular momentum of the rotating portion of the propulsion system
%
% DESCRIPTION: 
%   This function calculates the angular momentum and rate of angular
%   momentum components for the rotating portion of each propulsor. The
%   contributions from each propulsor are then summed to output the total
%   angular moment and angular momentum rate.
%
% INPUTS:
%   EngSpeed - Npx1 engine rotational speed [rad/s]
%   EngAccel - Npx1 engine rotational speed rate [rad/s^2]
%   Model - Model parameters
%
% OUTPUTS:
%   H_b - 3x1 total angular momentum in the body frame [slug-ft^2/s]
%   Hdot_b - 3x1 total angular momentum rate in the body frame [slug-ft^2/s^2]
%
% WRITTEN BY:
%   Benjamin M. Simmons
%   NASA Langley Research Center
%   Email: benjamin.m.simmons@nasa.gov
%
% HISTORY:
%   February 16, 2021 - Created and debugged, BMS
%

% propulsion inertia [slug-ft^2]
Ip=Model.Ip';

% unit vector of the propeller/rotor axis of rotation
p_rot_axis_e=Model.p_T_e;

% propeller/rotor rotation direction (CW=+1, CCW=-1)
Prop_dir=Model.prop_spin';

% hub frame angular momentum and angular momentum rate
H_h=EngSpeed.*Ip.*Prop_dir;
Hdot_h=EngAccel.*Ip.*Prop_dir;

% body frame angular momentum and angular momentum rate
H_b=p_rot_axis_e*H_h;
Hdot_b=p_rot_axis_e*Hdot_h;

% no angular momentum
% H_b=[0;0;0];
% Hdot_b=[0;0;0];

return
